simulink model "PlantWithTimeDelay"  (R2023b)
settings: Solver=VariableStepAuto  StartTime=0.0  StopTime=20.0  RelTol=1e-3
values from neighbouring files (symbols this model uses):
  G7_den = [a b c d e f]    [FirstOrderSystem_PlantWithTimeDelay.m]
  G7_num = [A B C D E]    [FirstOrderSystem_PlantWithTimeDelay.m]
settings Model: Creator=Zolo  LastModifiedBy=Zolo

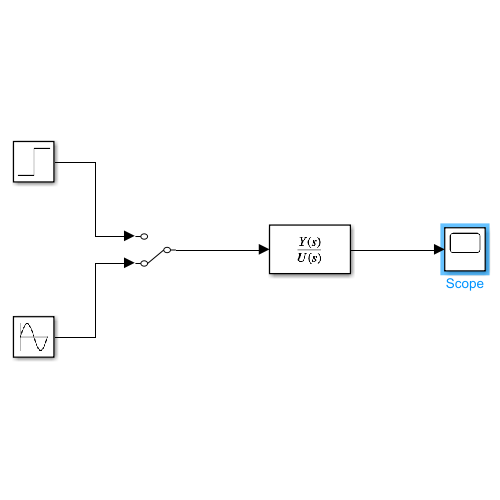
[thumbnail: Simulink's stored preview of the top-level diagram]
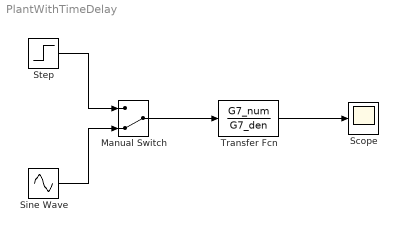
== system PlantWithTimeDelay ==
  Manual Switch : ManualSwitch  CurrentSetting=0
  Scope : Scope
  Sine Wave : Sin  SampleTime=0
  Step : Step  SampleTime=0
  Transfer Fcn : TransferFcn  Numerator=G7_num  Denominator=G7_den
  wires:
  Transfer Fcn/1 -> Scope/1
  Sine Wave/1 -> Manual Switch/2
  Step/1 -> Manual Switch/1
  Manual Switch/1 -> Transfer Fcn/1
